simulink model "Lab2EcommSim"  (R2020b)
settings: Solver=VariableStepAuto  StartTime=0.0  StopTime=10.0  RelTol=1e-3
model workspace (MAT data in the model file):
  tau = 0.0253302959106
libraries: simulink x1
settings Model: Creator=Jack  LastModifiedBy=Jack

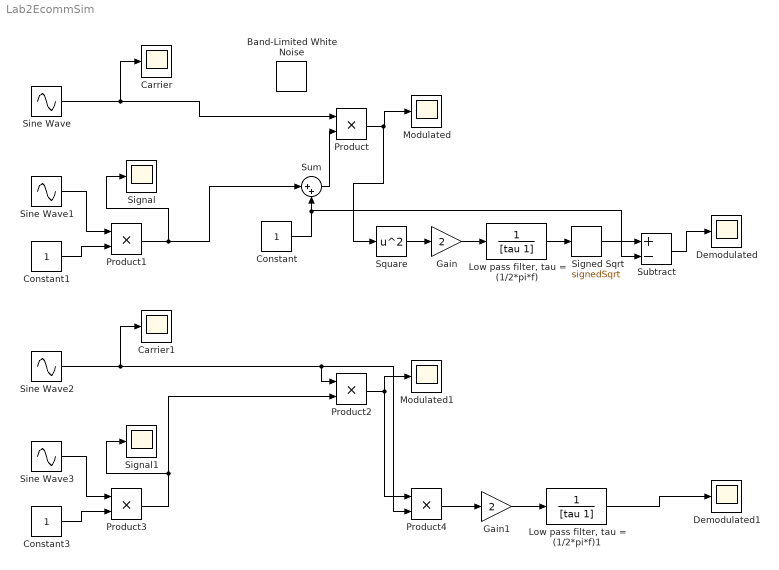
== system Lab2EcommSim ==
  Band-Limited White Noise : simulink/Sources/Band-Limited White Noise  Cov=[0.1]  Ts=1/5000  seed=[23341]
  Carrier : Scope
  Carrier1 : Scope
  Constant : Constant
  Constant1 : Constant
  Constant3 : Constant
  Demodulated : Scope
  Demodulated1 : Scope
  Gain : Gain  Gain=2
  Gain1 : Gain  Gain=2
  "Low pass filter, tau = (1/2*pi*f)" : TransferFcn  Denominator=[tau 1]
  "Low pass filter, tau = (1/2*pi*f)1" : TransferFcn  Denominator=[tau 1]
  Modulated : Scope
  Modulated1 : Scope
  Product{,1..4} (5 alike) : Product
  Signal : Scope
  Signal1 : Scope
  Signed Sqrt : Sqrt  Operator=signedSqrt  SaturateOnIntegerOverflow=on
  Sine Wave : Sin  Frequency=2*pi*25  SampleTime=1/5000
  Sine Wave1 : Sin  Frequency=2*pi  SampleTime=1/5000
  Sine Wave2 : Sin  Frequency=2*pi*25  SampleTime=1/5000
  Sine Wave3 : Sin  Frequency=2*pi  SampleTime=1/5000
  Square : Math  Operator=square  SaturateOnIntegerOverflow=on
  Subtract : Sum  Inputs=+-
  Sum : Sum  Inputs=|++
  wires:
  Constant1/1 -> Product1/2
  Sine Wave1/1 -> Product1/1
  Product1/1 -> Signal/1, Sum/1
  Constant/1 -> Subtract/2, Sum/2
  Sum/1 -> Product/2
  Product/1 -> Square/1, Modulated/1
  Sine Wave/1 -> Carrier/1, Product/1
  Gain/1 -> "Low pass filter, tau = (1/2*pi*f)"/1
  Signed Sqrt/1 -> Subtract/1
  "Low pass filter, tau = (1/2*pi*f)"/1 -> Signed Sqrt/1
  Square/1 -> Gain/1
  Subtract/1 -> Demodulated/1
  "Low pass filter, tau = (1/2*pi*f)1"/1 -> Demodulated1/1
  Product3/1 -> Product2/2, Signal1/1
  Sine Wave2/1 -> Carrier1/1, Product4/2, Product2/1
  Sine Wave3/1 -> Product3/1
  Product2/1 -> Product4/1, Modulated1/1
  Constant3/1 -> Product3/2
  Product4/1 -> Gain1/1
  Gain1/1 -> "Low pass filter, tau = (1/2*pi*f)1"/1
